simulink model "digital_modulation"  (R2023a)
settings: Solver=VariableStepAuto  StartTime=0.0  StopTime=0.1  RelTol=1e-3
libraries: dspfdesign x2, commdigbbndpm3 x2, commchan3 x1, commrandsrc3 x1
settings Model: NumberOfSteps=20  Creator=tanov  LastModifiedBy=tanov

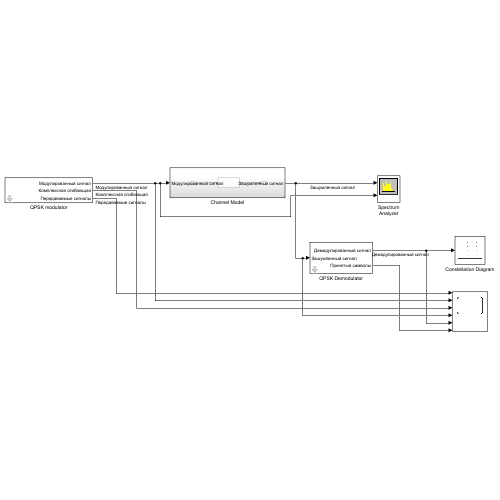
[thumbnail: Simulink's stored preview of the top-level diagram]
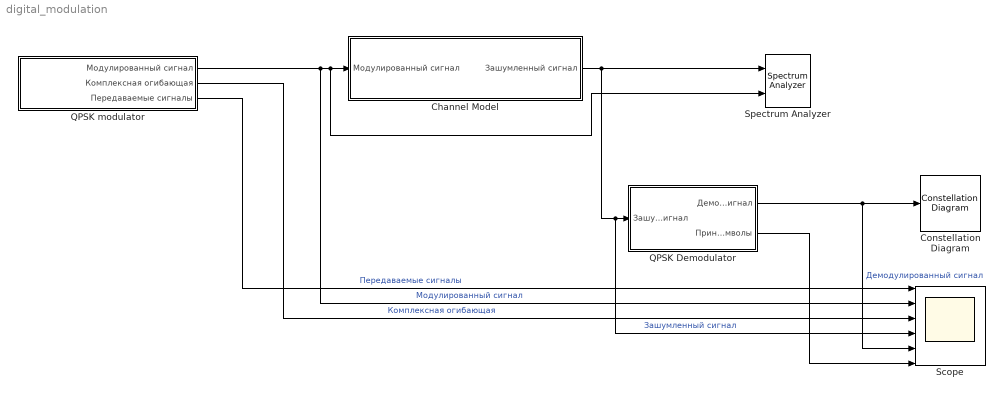
== system digital_modulation ==
  Channel Model : Subsystem
  Constellation Diagram : ConstellationDiagram  WindowPosition=[1.000000,49.000000,1600.000000,930.000000,]  ScopeFrameLocation=window  SamplesPerSymbol=100  SymbolsToDisplaySource=Property  SymbolsToDisplay=300  XLimits=[-1.46,1.46]  YLimits=[-1.38,1.38]  ShowLegend=on  DefaultConfigurationName=comm.scopes.ConstellationDiagramBlockCfg
  QPSK Demodulator : Subsystem  mask{SR=1000, f_c=10000, f_d=100000}
      mask prompts: SR "Символьная скорость, симв/сек"; f_c "Частота несущей, Гц"; f_d "Частота дискретизации, Гц"
  QPSK modulator : Subsystem  mask{SR=10000, f_c=1000, f_d=100}
      mask prompts: SR "Символьная скорость, симв/сек"; f_c "Частота несущей, Гц"; f_d "Частота дискретизации, Гц"
  Scope : Scope  NumInputPorts=6
  Spectrum Analyzer : SpectrumAnalyzer  NumInputPorts=2  WindowPosition=[1.000000,49.000000,1600.000000,930.000000,]  ScopeFrameLocation=window  YLimits=[-71.78054219,15.01686381]  ColorLimits=[-20 80]  ShowLegend=on  DefaultConfigurationName=spbscopes.SpectrumAnalyzerBlockCfg  IsFrequencyInputMode=0  FrequencyVectorPort=0  FrequencyVectorFromPort=0  FrequencyInputRBWPort=0  FrequencyInputRBWFromPort=0
  wires:
  QPSK modulator/1(Модулированный сигнал) -> Scope/2, Spectrum Analyzer/2, Channel Model/1(Модулированный сигнал)  "Модулированный сигнал"
  Channel Model/1(Зашумленный сигнал) -> Scope/4, QPSK Demodulator/1(Зашумленный сигнал), Spectrum Analyzer/1  "Зашумленный сигнал"
  QPSK Demodulator/1(Демодулированный сигнал) -> Constellation Diagram/1, Scope/5  "Демодулированный сигнал"
  QPSK modulator/3(Передаваемые сигналы) -> Scope/1  "Передаваемые сигналы"
  QPSK modulator/2(Комплексная огибающая) -> Scope/3  "Комплексная огибающая"
  QPSK Demodulator/2(Принятые символы) -> Scope/6

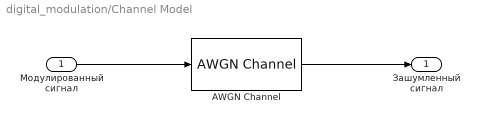
== system digital_modulation/Channel Model ==
  Модулированный сигнал : Inport
  AWGN Channel : commchan3/AWGN Channel  LegacyMode=off  NoiseMethod="Signal to noise ratio  (SNR)"  noiseMode="Signal to noise ratio  (SNR)"  EbNo=10  EsNo=10  SNR=20  BitsPerSymbol=1  SignalPower=1  SamplesPerSymbol=1  SymbolPeriod=1  VarianceSource=Parameter  Variance=1  RandomStream=Global stream  Seed=67  SimulateUsing=Code generation
  Зашумленный сигнал : Outport
  wires:
  AWGN Channel/1 -> Зашумленный сигнал/1
  Модулированный сигнал/1 -> AWGN Channel/1

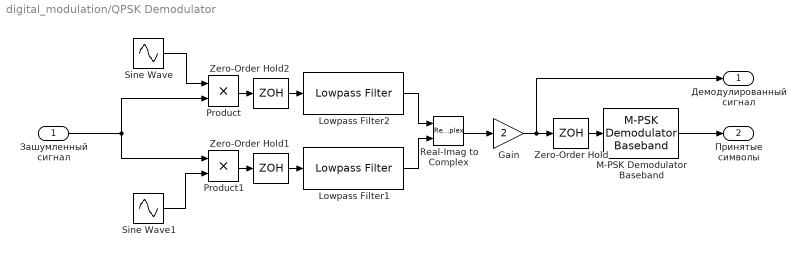
== system digital_modulation/QPSK Demodulator ==
  Зашумленный сигнал : Inport
  Gain : Gain  Gain=2
  Lowpass Filter1 : dspfdesign/Lowpass Filter  FilterType=FIR  DesignForMinimumOrder=on  FilterOrder=50  PassbandFrequency=8e3  StopbandFrequency=12e3  PassbandRipple=0.1  StopbandAttenuation=80  SampleRateMode=Specify on dialog  SampleRate=44100  SimulateUsing=Interpreted execution  roundingMode=Floor  coeffsDataTypeStr=fixdt(1,16)
  Lowpass Filter2 : dspfdesign/Lowpass Filter  FilterType=FIR  DesignForMinimumOrder=on  FilterOrder=50  PassbandFrequency=8e3  StopbandFrequency=12e3  PassbandRipple=0.1  StopbandAttenuation=80  SampleRateMode=Specify on dialog  SampleRate=44100  SimulateUsing=Interpreted execution  roundingMode=Floor  coeffsDataTypeStr=fixdt(1,16)
  M-PSK Demodulator Baseband : commdigbbndpm3/M-PSK Demodulator Baseband  M=8  OutType=Integer  DecType=Hard decision  VarSource=Dialog  Variance=1  Dec=Gray  Mapping=[0:7]  Ph=pi/4  outDtype1=Inherit via internal rule  outDtype2=Inherit via internal rule  derotateFactorWordLen=16  derotateFactorDataTypeStr=Inherit: Same word length as input  derotateFactorLastDataTypeStr=Inherit: Same word length as input
  Product : Product
  Product1 : Product
  Real-Imag to Complex : RealImagToComplex
  Sine Wave : Sin  Frequency=2*pi*f_c  SampleTime=0
  Sine Wave1 : Sin  Frequency=2*pi*f_c  Phase=pi/2  SampleTime=0
  Zero-Order Hold : ZeroOrderHold  SampleTime=1e-3
  Zero-Order Hold1 : ZeroOrderHold  SampleTime=(1/f_c)/10
  Zero-Order Hold2 : ZeroOrderHold  SampleTime=(1/f_c)/10
  Демодулированный сигнал : Outport
  Принятые символы : Outport  Port=2
  wires:
  Зашумленный сигнал/1 -> Product1/1, Product/2
  Sine Wave/1 -> Product/1
  Sine Wave1/1 -> Product1/2
  Real-Imag to Complex/1 -> Gain/1
  Lowpass Filter2/1 -> Real-Imag to Complex/1
  Lowpass Filter1/1 -> Real-Imag to Complex/2
  Gain/1 -> Демодулированный сигнал/1, Zero-Order Hold/1
  Zero-Order Hold/1 -> M-PSK Demodulator Baseband/1
  M-PSK Demodulator Baseband/1 -> Принятые символы/1
  Product1/1 -> Zero-Order Hold1/1
  Zero-Order Hold1/1 -> Lowpass Filter1/1
  Product/1 -> Zero-Order Hold2/1
  Zero-Order Hold2/1 -> Lowpass Filter2/1

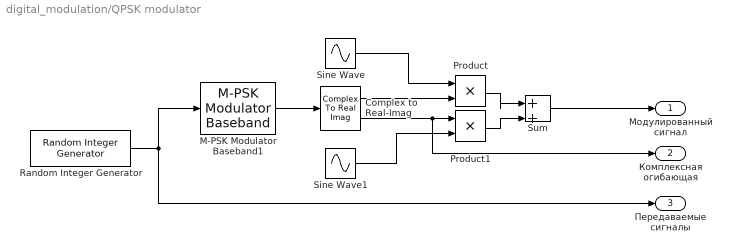
== system digital_modulation/QPSK modulator ==
  Complex to Real-Imag : ComplexToRealImag
  M-PSK Modulator Baseband1 : commdigbbndpm3/M-PSK Modulator Baseband  M=8  InType=Integer  Enc=Gray  Mapping=[0:7]  Ph=pi/4  outDtype=double  outWordLen=16  outUDDataType=sfix(16)  outFracLenMode=Best precision  outFracLen=15  outDataTypeStr=double  outLastDataTypeStr=double
      settings: LibrarySourceBlock=|
      | commhdldigbbndpm/M-PSK
      | Modulator
      | Baseband
  Product : Product
  Product1 : Product
  Random Integer Generator : commrandsrc3/Random Integer Generator  SetSize=8  SeedSource=Auto  Seed=0  SampleTime=1/SR  SamplesPerFrame=1  OutputDataType=double  SimulateUsing=Interpreted execution
  Sine Wave : Sin  Frequency=2*pi*f_c  Phase=-pi/4  SampleTime=2*pi*f_d
  Sine Wave1 : Sin  Frequency=2*pi*f_c  Phase=pi/4  SampleTime=2*pi*f_d
  Sum : Sum  Inputs=|++
  Модулированный сигнал : Outport
  Комплексная огибающая : Outport  Port=2
  Передаваемые сигналы : Outport  Port=3
  wires:
  Random Integer Generator/1 -> M-PSK Modulator Baseband1/1, Передаваемые сигналы/1
  M-PSK Modulator Baseband1/1 -> Complex to Real-Imag/1
  Complex to Real-Imag/1 -> Product/2
  Sine Wave/1 -> Product/1
  Complex to Real-Imag/2 -> Комплексная огибающая/1, Product1/1
  Sine Wave1/1 -> Product1/2
  Product/1 -> Sum/1
  Product1/1 -> Sum/2
  Sum/1 -> Модулированный сигнал/1
